simulink model "cycletest_3d"  (R2023a)
settings: Solver=ode1  StartTime=0.0  StopTime=400  FixedStep=0.002  RelTol=1e-3  EnableMultiTasking=on
values from neighbouring files (symbols this model uses):
  beta3d = 0.9    [loadResultData.m]    (also in simulate_hover.m; temp.m)
  cycleGain = 0.2    [simulate_hover.m]    (also in temp.m = 1)
  epsilon3d = 1    [loadResultData.m]    (also in simulate_hover.m; temp.m)
  Jp = 2*Jeq_prop    (= 0.0552224595625)    [setup_lab_hover.m]    (also in simulate_hover.m)
  Jr = 2*Jeq_prop    (= 0.0552224595625)    [setup_lab_hover.m]    (also in simulate_hover.m)
  Jy = 4*Jeq_prop    (= 0.110444919125)    [setup_lab_hover.m]    (also in simulate_hover.m)
  K = lqi(sys, Q, R)    [simulate_hover.m]
  k3d = 1.65    [loadResultData.m]    (also in simulate_hover.m; temp.m)
  Kf = 0.1188    [setup_lab_hover.m]    (also in simulate_hover.m)
  Kt = 0.0036    [setup_lab_hover.m]    (also in simulate_hover.m)
  L = 7.75*0.0254    (= 0.19685)    [setup_lab_hover.m]    (also in simulate_hover.m = 0.1969)
  sigma = 0    [simulate_hover.m]
  velMax = 100*60*pi/180    (= 104.71975512)    [simulate_hover.m]
  VMAX_AMP = 24    [setup_lab_hover.m]    (also in simulate_hover.m)
  wcf = 2 * pi * 20    (= 125.663706144)    [setup_lab_hover.m]    (also in simulate_hover.m)
  zetaf = 0.6    [setup_lab_hover.m]    (also in simulate_hover.m)
libraries: simulink_extras x1, dspsrcs4 x1
settings Model: ExtModeTrigDuration=10000  Creator=kille  LastModifiedBy=Jacob
settings SolverCC: AlgebraicLoopSolver=TrustRegion  PositivePriorityOrder=on  AutoInsertRateTranBlk=on
settings DataIOCC: ReturnWorkspaceOutputs=off
settings OptimizationCC: LifeSpan=inf
settings DebuggingCC: UnconnectedInputMsg=warning  UnconnectedOutputMsg=warning  UnconnectedLineMsg=warning  ArithmeticOperatorsInVariantConditions=warning
settings ModelReferenceCC: EnableRefExpFcnMdlSchedulingChecks=on
settings SFSimCC: SimUseLocalCustomCode=off  CustomCodeUndefinedFunction=UseInterfaceOnly
settings RTWCC: Description=QUARC Win64 Target  SystemTargetFile=quarc_win64.tlc  TemplateMakefile=quarc_default_tmf  RTWUseLocalCustomCode=off
settings CodeAppCC: StateflowObjectComments=on
settings STFCustomTargetCC: TargetPreCompLibLocation=C:\PROGRA~3\QUARC\lib\2016a\win64\release  UseToolchainInfoCompliant=off  SystemTargetFile=quarc_win64.tlc
settings GRTTargetCC: TargetPreCompLibLocation=C:\PROGRA~3\QUARC\lib\2016a\win64\release  ParMdlRefBuildCompliant=off  CompOptLevelCompliant=off  CombineOutputUpdateFcns=off  MatFileLogging=off  CPPClassGenCompliant=off  GRTInterface=on  UseToolchainInfoCompliant=off  ExtMode=on  ExtModeMexFile=quarc_comm
settings ConfigComp: CovMetricSettings=dswe

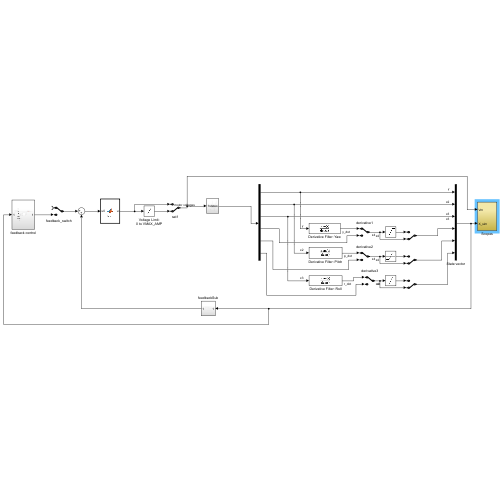
[thumbnail: Simulink's stored preview of the top-level diagram]
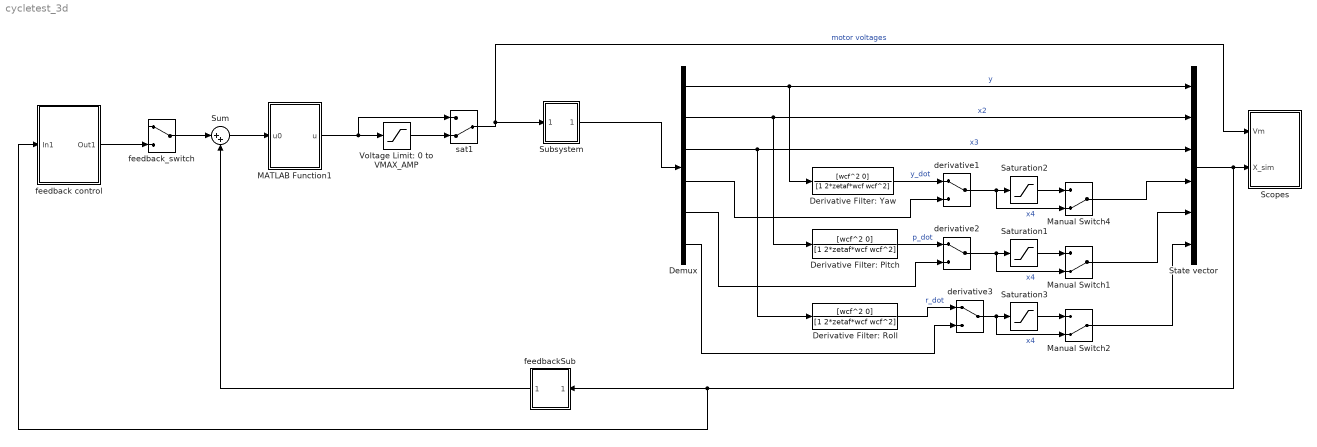
== system cycletest_3d ==
  Demux : Demux  Outputs=6
  Derivative Filter: Pitch : TransferFcn  Numerator=[wcf^2 0]  Denominator=[1 2*zetaf*wcf wcf^2]
  Derivative Filter: Roll : TransferFcn  Numerator=[wcf^2 0]  Denominator=[1 2*zetaf*wcf wcf^2]
  Derivative Filter: Yaw : TransferFcn  Numerator=[wcf^2 0]  Denominator=[1 2*zetaf*wcf wcf^2]
  MATLAB Function1 : MATLAB Function  TreatAsAtomicUnit=on
  Manual Switch1 : ManualSwitch  CurrentSetting=0
  Manual Switch2 : ManualSwitch  CurrentSetting=0
  Manual Switch4 : ManualSwitch  CurrentSetting=0
  Saturation1 : Saturate  UpperLimit=velMax  LowerLimit=-velMax
  Saturation2 : Saturate  UpperLimit=velMax  LowerLimit=-velMax
  Saturation3 : Saturate  UpperLimit=velMax  LowerLimit=-velMax
  Scopes : Subsystem
  State vector : Mux  Inputs=6
  Subsystem : Subsystem
  Sum : Sum  Inputs=|++
  Voltage Limit: 0 to VMAX_AMP : Saturate  UpperLimit=VMAX_AMP  LowerLimit=0
  derivative1 : ManualSwitch
  derivative2 : ManualSwitch
  derivative3 : ManualSwitch
  feedback control : Subsystem
  feedbackSub : Subsystem
  feedback_switch : ManualSwitch
  sat1 : ManualSwitch  CurrentSetting=0
  wires:
  Demux/1 -> State vector/1, Derivative Filter: Yaw/1  "y"
  sat1/1 -> Scopes/1(Vm), Subsystem/1(Input)  "motor voltages"
  Derivative Filter: Yaw/1 -> derivative1/1  "y_dot"
  Demux/4 -> derivative1/2
  Derivative Filter: Pitch/1 -> derivative2/1  "p_dot"
  Derivative Filter: Roll/1 -> derivative3/1  "r_dot"
  Demux/5 -> derivative2/2
  Demux/6 -> derivative3/2
  derivative1/1 -> Manual Switch4/2, Saturation2/1  "x4"
  Saturation2/1 -> Manual Switch4/1
  derivative2/1 -> Manual Switch1/2, Saturation1/1  "x4"
  Saturation1/1 -> Manual Switch1/1
  derivative3/1 -> Manual Switch2/2, Saturation3/1  "x4"
  Saturation3/1 -> Manual Switch2/1
  Manual Switch4/1 -> State vector/4
  Manual Switch1/1 -> State vector/5
  Manual Switch2/1 -> State vector/6
  Demux/3 -> State vector/3, Derivative Filter: Roll/1  "x3"
  Demux/2 -> State vector/2, Derivative Filter: Pitch/1  "x2"
  Subsystem/1(states) -> Demux/1
  Voltage Limit: 0 to VMAX_AMP/1 -> sat1/2
  MATLAB Function1/1(u) -> sat1/1, Voltage Limit: 0 to VMAX_AMP/1
  Sum/1 -> MATLAB Function1/1(u0)
  State vector/1 -> feedback control/1(In1), feedbackSub/1(Input), Scopes/2(X_sim)
  feedback control/1(Out1) -> feedback_switch/2
  feedback_switch/1 -> Sum/1
  feedbackSub/1(Out1) -> Sum/2

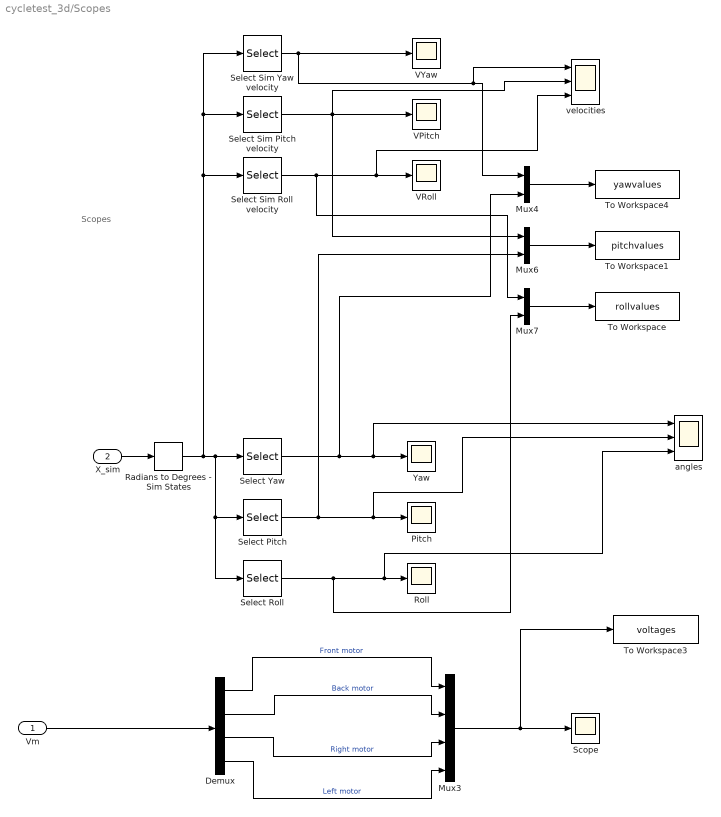
== system cycletest_3d/Scopes ==
  note: Scopes
  Vm : Inport
  X_sim : Inport  Port=2
  Demux : Demux
  Mux3 : Mux
  Mux4 : Mux  Inputs=2
  Mux6 : Mux  Inputs=2
  Mux7 : Mux  Inputs=2
  Pitch : Scope
  Radians to Degrees - Sim States : simulink_extras/Transformations/Radians to Degrees
  Roll : Scope
  Scope : Scope
  Select Pitch : Selector  InputPortWidth=6  IndexOptions=Index vector (dialog)  Indices=2  OutputSizes=1
  Select Roll : Selector  InputPortWidth=6  IndexOptions=Index vector (dialog)  Indices=3  OutputSizes=1
  Select Sim Pitch velocity : Selector  InputPortWidth=6  IndexOptions=Index vector (dialog)  Indices=5  OutputSizes=1
  Select Sim Roll velocity : Selector  InputPortWidth=6  IndexOptions=Index vector (dialog)  Indices=6  OutputSizes=1
  Select Sim Yaw velocity : Selector  InputPortWidth=6  IndexOptions=Index vector (dialog)  Indices=4  OutputSizes=1
  Select Yaw : Selector  InputPortWidth=6  IndexOptions=Index vector (dialog)  Indices=1  OutputSizes=1
  To Workspace : ToWorkspace  VariableName=rollvalues  SampleTime=-1
  To Workspace1 : ToWorkspace  VariableName=pitchvalues  SampleTime=-1
  To Workspace3 : ToWorkspace  VariableName=voltages  SampleTime=-1
  To Workspace4 : ToWorkspace  VariableName=yawvalues  SampleTime=-1
  VPitch : Scope
  VRoll : Scope
  VYaw : Scope
  Yaw : Scope
  angles : Scope  NumInputPorts=3
  velocities : Scope  NumInputPorts=3
  wires:
  Select Roll/1 -> angles/3, Roll/1, Mux7/2
  Radians to Degrees - Sim States/1 -> Select Sim Roll velocity/1, Select Sim Pitch velocity/1, Select Sim Yaw velocity/1, Select Roll/1, Select Pitch/1, Select Yaw/1
  Select Pitch/1 -> angles/2, Pitch/1, Mux6/2
  X_sim/1 -> Radians to Degrees - Sim States/1
  Demux/1 -> Mux3/1  "Front motor"
  Demux/2 -> Mux3/2  "Back motor"
  Demux/3 -> Mux3/3  "Right motor"
  Demux/4 -> Mux3/4  "Left motor"
  Vm/1 -> Demux/1
  Select Sim Yaw velocity/1 -> VYaw/1, velocities/1, Mux4/1
  Select Sim Roll velocity/1 -> velocities/3, VRoll/1, Mux7/1
  Select Sim Pitch velocity/1 -> Mux6/1, velocities/2, VPitch/1
  Mux4/1 -> To Workspace4/1
  Mux6/1 -> To Workspace1/1
  Mux7/1 -> To Workspace/1
  Mux3/1 -> To Workspace3/1, Scope/1
  Select Yaw/1 -> angles/1, Yaw/1, Mux4/2

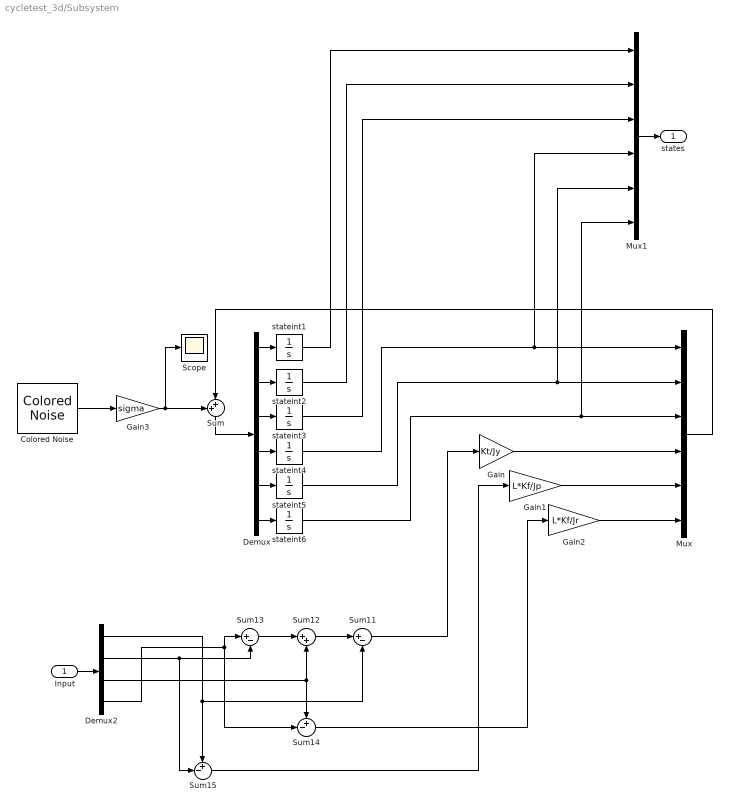
== system cycletest_3d/Subsystem ==
  Input : Inport
  Colored Noise : dspsrcs4/Colored Noise  Color=white  InverseFrequencyPower=1  BoundedOutput=off  NumChannels=6  OutputDataType=double  SamplesPerFrame=1  SampleTime=1  RandomStream=mt19937ar with seed  Seed=67  SimulateUsing=Interpreted execution
  Demux : Demux  Outputs=6
  Demux2 : Demux
  Gain : Gain  Gain=Kt/Jy
  Gain1 : Gain  Gain=L*Kf/Jp
  Gain2 : Gain  Gain=L*Kf/Jr
  Gain3 : Gain  Gain=sigma
  Mux : Mux  Inputs=6
  Mux1 : Mux  Inputs=6
  Scope : Scope
  Sum : Sum  Inputs=++|
  Sum11 : Sum  Inputs=|+-
  Sum12 : Sum  Inputs=|++
  Sum13 : Sum  Inputs=|+-
  Sum14 : Sum  Inputs=+-|
  Sum15 : Sum  Inputs=+-|
  stateint{1,4..6} (4 alike) : Integrator
  stateint2 : Integrator  InitialCondition=0.00010472
  stateint3 : Integrator  InitialCondition=0.00010472
  states : Outport
  wires:
  stateint5/1 -> Mux/2, Mux1/5
  Gain2/1 -> Mux/6
  Gain1/1 -> Mux/5
  stateint6/1 -> Mux/3, Mux1/6
  stateint4/1 -> Mux/1, Mux1/4
  Gain/1 -> Mux/4
  Mux/1 -> Sum/2
  Gain3/1 -> Scope/1, Sum/1
  Demux2/4 -> Sum13/1, Sum14/2
  Demux2/1 -> Sum15/1, Sum11/2
  Demux2/2 -> Sum13/2, Sum15/2
  Sum12/1 -> Sum11/1
  Sum11/1 -> Gain/1
  Demux2/3 -> Sum12/2, Sum14/1
  Sum13/1 -> Sum12/1
  Input/1 -> Demux2/1
  Sum/1 -> Demux/1
  Demux/1 -> stateint1/1
  Demux/2 -> stateint2/1
  Demux/3 -> stateint3/1
  Demux/4 -> stateint4/1
  Demux/5 -> stateint5/1
  Demux/6 -> stateint6/1
  Mux1/1 -> states/1
  stateint1/1 -> Mux1/1
  stateint2/1 -> Mux1/2
  stateint3/1 -> Mux1/3
  Sum15/1 -> Gain1/1
  Sum14/1 -> Gain2/1
  Colored Noise/1 -> Gain3/1

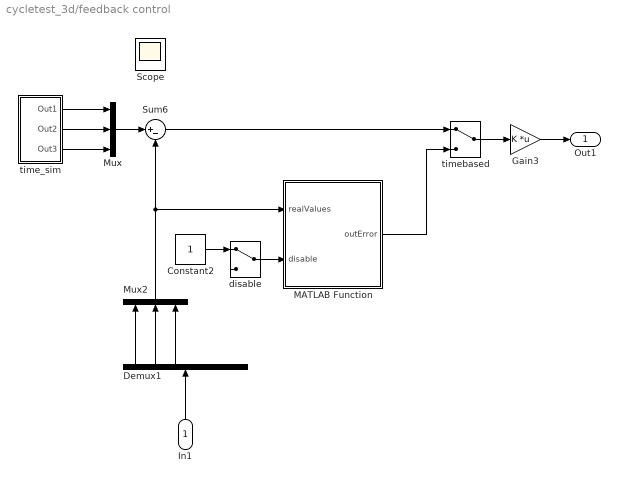
== system cycletest_3d/feedback control ==
  In1 : Inport
  Constant2 : Constant
  Demux1 : Demux  Outputs=6
  Gain3 : Gain  Gain=K  Multiplication=Matrix(K*u)
  MATLAB Function : MATLAB Function  TreatAsAtomicUnit=on
  Mux : Mux  Inputs=3
  Mux2 : Mux  Inputs=3
  Scope : Scope
  Sum6 : Sum  Inputs=|+-
  disable : ManualSwitch
  time_sim : Subsystem
  timebased : ManualSwitch
  Out1 : Outport
  wires:
  Demux1/2 -> Mux2/2
  Demux1/1 -> Mux2/1
  Demux1/3 -> Mux2/3
  In1/1 -> Demux1/1
  MATLAB Function/1(outError) -> timebased/2
  Sum6/1 -> timebased/1
  timebased/1 -> Gain3/1
  Gain3/1 -> Out1/1
  Mux2/1 -> Sum6/2, MATLAB Function/1(realValues)
  disable/1 -> MATLAB Function/2(disable)
  Constant2/1 -> disable/1
  Mux/1 -> Sum6/1
  time_sim/1(Out1) -> Mux/1
  time_sim/2(Out2) -> Mux/2
  time_sim/3(Out3) -> Mux/3

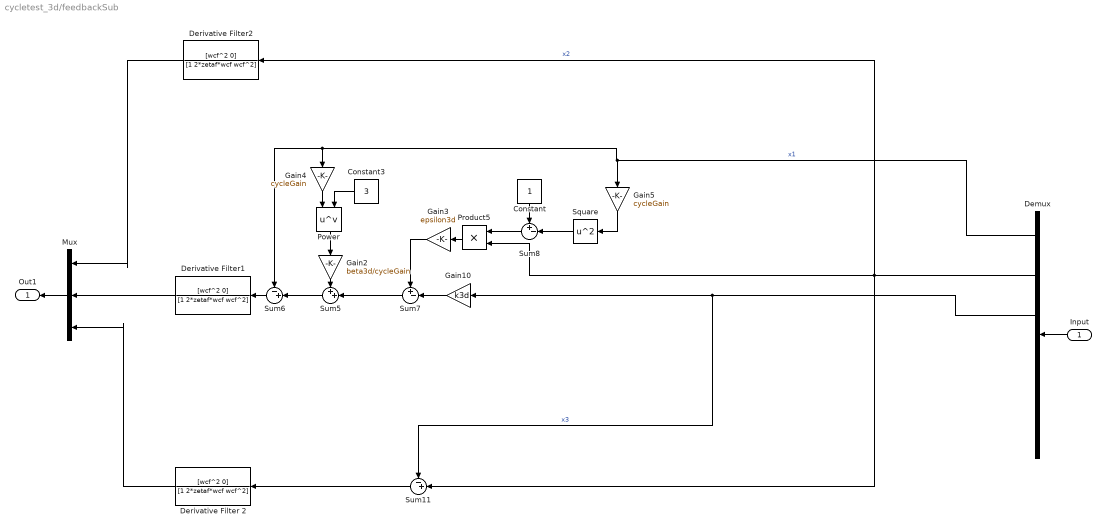
== system cycletest_3d/feedbackSub ==
  Input : Inport
  Constant : Constant
  Constant3 : Constant  Value=3
  Demux : Demux  Outputs=6
  Derivative Filter 2 : TransferFcn  Numerator=[wcf^2 0]  Denominator=[1 2*zetaf*wcf wcf^2]
  Derivative Filter1 : TransferFcn  Numerator=[wcf^2 0]  Denominator=[1 2*zetaf*wcf wcf^2]
  Derivative Filter2 : TransferFcn  Numerator=[wcf^2 0]  Denominator=[1 2*zetaf*wcf wcf^2]
  Gain10 : Gain  Gain=k3d
  Gain2 : Gain  Gain=beta3d/cycleGain
  Gain3 : Gain  Gain=epsilon3d
  Gain4 : Gain  Gain=cycleGain
  Gain5 : Gain  Gain=cycleGain
  Mux : Mux  Inputs=3
  Power : Math  Operator=pow
  Product5 : Product
  Square : Math  Operator=square
  Sum11 : Sum  Inputs=-+|
  Sum5 : Sum  Inputs=++|
  Sum6 : Sum  Inputs=-+|
  Sum7 : Sum  Inputs=+-|
  Sum8 : Sum  Inputs=+-|
  Out1 : Outport
  wires:
  Input/1 -> Demux/1
  Sum7/1 -> Sum5/2
  Sum5/1 -> Sum6/2
  Gain4/1 -> Power/1
  Demux/1 -> Gain4/1, Sum6/1, Gain5/1  "x1"
  Gain5/1 -> Square/1
  Product5/1 -> Gain3/1
  Sum6/1 -> Derivative Filter1/1
  Power/1 -> Gain2/1
  Constant3/1 -> Power/2
  Gain10/1 -> Sum7/2
  Constant/1 -> Sum8/1
  Sum8/1 -> Product5/1
  Square/1 -> Sum8/2
  Gain2/1 -> Sum5/1
  Gain3/1 -> Sum7/1
  Sum11/1 -> Derivative Filter 2/1
  Demux/3 -> Sum11/1, Gain10/1  "x3"
  Demux/2 -> Derivative Filter2/1, Product5/2, Sum11/2  "x2"
  Derivative Filter2/1 -> Mux/1
  Derivative Filter1/1 -> Mux/2
  Derivative Filter 2/1 -> Mux/3
  Mux/1 -> Out1/1

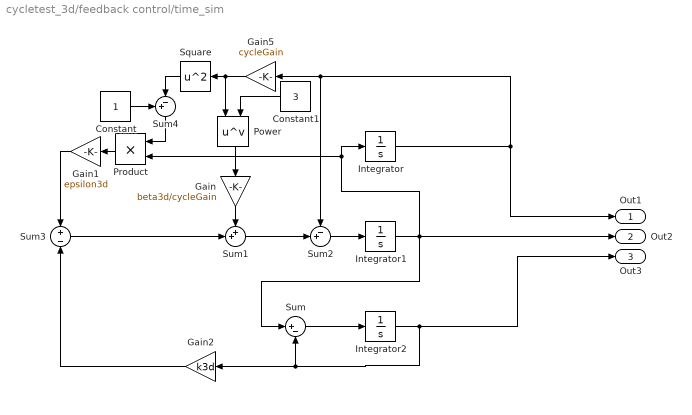
== system cycletest_3d/feedback control/time_sim ==
  Constant : Constant
  Constant1 : Constant  Value=3
  Gain : Gain  Gain=beta3d/cycleGain
  Gain1 : Gain  Gain=epsilon3d
  Gain2 : Gain  Gain=k3d
  Gain5 : Gain  Gain=cycleGain
  Integrator : Integrator  InitialCondition=0.0001
  Integrator1 : Integrator  InitialCondition=0.0001
  Integrator2 : Integrator  InitialCondition=0.0001
  Power : Math  Operator=pow
  Product : Product
  Square : Math  Operator=square
  Sum : Sum  Inputs=|+-
  Sum1 : Sum  Inputs=++|
  Sum2 : Sum  Inputs=-+|
  Sum3 : Sum  Inputs=+|-
  Sum4 : Sum  Inputs=+-|
  Out1 : Outport
  Out2 : Outport  Port=2
  Out3 : Outport  Port=3
  wires:
  Gain5/1 -> Square/1, Power/1
  Integrator1/1 -> Out2/1, Sum/1, Product/2, Integrator/1
  Constant/1 -> Sum4/1
  Integrator2/1 -> Out3/1, Sum/2, Gain2/1
  Gain/1 -> Sum1/1
  Square/1 -> Sum4/2
  Integrator/1 -> Out1/1, Sum2/1, Gain5/1
  Sum2/1 -> Integrator1/1
  Sum1/1 -> Sum2/2
  Power/1 -> Gain/1
  Sum4/1 -> Product/1
  Sum3/1 -> Sum1/2
  Sum/1 -> Integrator2/1
  Gain1/1 -> Sum3/1
  Constant1/1 -> Power/2
  Product/1 -> Gain1/1
  Gain2/1 -> Sum3/2

== matlab function cycletest_3d/feedback control/MATLAB Function ==
  data: realValues input; outError output; disable input
function outError = approxLimitSimu(realValues, disable)
    outError = transpose([0, 0, 0]);
    %temp = load('paperCycle.mat');
    %cycleValues = temp.paperCycle;
    %for n = 1:2
    %    cycleN = cycleValues(:, n);
    %    realValueN = realValues(n);
    %    [closestValueError,idx]=min(abs(cycleN-realValueN));
    %    outError(n) = closestValueError;
    %end
    %disp(length(cycleValues))
    coder.extrinsic('approxLimit');
    if disable ~= 1
        outError = transpose(approxLimit(realValues));
    end

== matlab function cycletest_3d/MATLAB Function1 ==
  data: u output; u0 input
function u = fcn(u0)
    % %x1, x2, x3, x4, x5, x6 = x;
    % uG1 = 0;
    % uG2 = 0;
    u1 = 0;
    u2 = 0;
    u3 = 0;
    u4 = 0;

    coder.extrinsic('solveSyms3d_3');
    % coder.extrinsic('solveSyms4');
    % if x5 ~= 0 & x6 ~= 0
    %     [u1, u2, u3, u4] = solveSyms4(x5, x6, u0(1), u0(2), u0(3));
    % else
    %     u1 = 0.01;
    %     u2 = 0.01;
    %     u3 = 0.01;
    %     u4 = 0.01;
    % 
    % end
    [u1, u2, u3, u4] = solveSyms3d_3(u0(1), u0(2), u0(3));
    u = transpose([u1 + 12, u2 + 12, u3 + 12, u4 + 12]);
    %u = transpose([u1, 12, u2, 12]);


end
